simulink model "pool_task"  (Simulink 3.00)
libraries: logiclib x14, mathlib x13, genlib x2, execlib x2, timelib x1

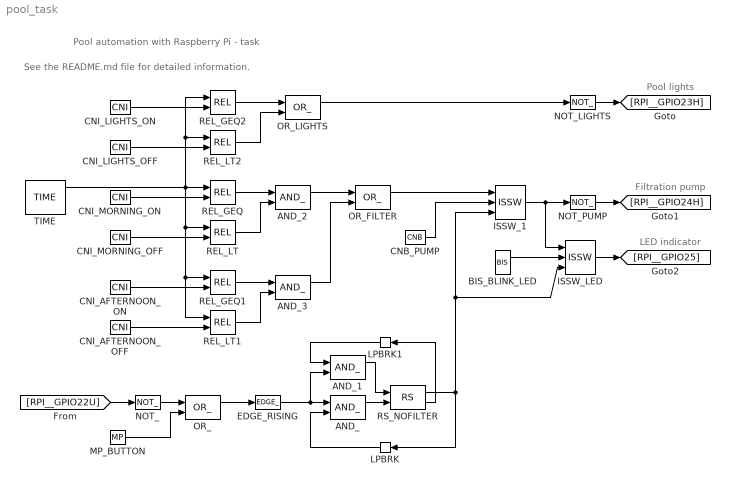
== system pool_task ==
  note: Pool lights
  note: Filtration pump
  note: LED indicator
  note: See the README.md file for detailed information.
  note: Pool automation with Raspberry Pi - task
  AND_{,1..3} (4 alike) : logiclib/AND_
  BIS_BLINK_LED : genlib/BIS  Y0=off  t1=0.1  t2=0.2  t3=0  t4=0  t5=0  t6=0  t7=2.0  t8=0  RPT=on  bEdit=off
  CNB_PUMP : mathlib/CNB  YCN=off
  CNI_AFTERNOON_OFF : mathlib/CNI  icn=14
  CNI_AFTERNOON_ON : mathlib/CNI  icn=13
  CNI_LIGHTS_OFF : mathlib/CNI  icn=1
  CNI_LIGHTS_ON : mathlib/CNI  icn=21
  CNI_MORNING_OFF : mathlib/CNI  icn=4
  CNI_MORNING_ON : mathlib/CNI  icn=2
  EDGE_RISING : logiclib/EDGE_  iedge=1: Rising edge
  ISSW_1 : logiclib/ISSW
  ISSW_LED : logiclib/ISSW
  LPBRK : execlib/LPBRK  Orientation=left
  LPBRK1 : execlib/LPBRK  Orientation=left
  MP_BUTTON : genlib/MP  pwidth=1  BSTATE=off  RPTF=off
  NOT_ : logiclib/NOT_
  NOT_LIGHTS : logiclib/NOT_
  NOT_PUMP : logiclib/NOT_
  OR_ : logiclib/OR_
  OR_FILTER : logiclib/OR_
  OR_LIGHTS : logiclib/OR_
  REL_GEQ : mathlib/REL  irel=6: greater or equal (>=)
  REL_GEQ1 : mathlib/REL  irel=6: greater or equal (>=)
  REL_GEQ2 : mathlib/REL  irel=6: greater or equal (>=)
  REL_LT : mathlib/REL  irel=3: less than (<)
  REL_LT1 : mathlib/REL  irel=3: less than (<)
  REL_LT2 : mathlib/REL  irel=3: less than (<)
  RS_NOFILTER : logiclib/RS
  TIME : timelib/TIME  tz=1: Local time
  wires:
  AND_/1 -> RS_NOFILTER/2
  AND_1/1 -> RS_NOFILTER/1
  AND_2/1 -> OR_FILTER/1
  AND_3/1 -> OR_FILTER/2
  BIS_BLINK_LED/1 -> ISSW_LED/2
  CNB_PUMP/1 -> ISSW_1/2
  CNI_AFTERNOON_OFF/1 -> REL_LT1/2
  CNI_AFTERNOON_ON/1 -> REL_GEQ1/2
  CNI_LIGHTS_OFF/1 -> REL_LT2/2
  CNI_LIGHTS_ON/1 -> REL_GEQ2/2
  CNI_MORNING_OFF/1 -> REL_LT/2
  CNI_MORNING_ON/1 -> REL_GEQ/2
  EDGE_RISING/1 -> AND_/1, AND_1/2
  [RPI__GPIO22U] -> NOT_/1
  ISSW_1/1 -> ISSW_LED/1, NOT_PUMP/1
  ISSW_LED/1 -> [RPI__GPIO25]
  LPBRK/1 -> AND_/2
  LPBRK1/1 -> AND_1/1
  MP_BUTTON/1 -> OR_/2
  NOT_/1 -> OR_/1
  NOT_LIGHTS/1 -> [RPI__GPIO23H]
  NOT_PUMP/1 -> [RPI__GPIO24H]
  OR_/1 -> EDGE_RISING/1
  OR_FILTER/1 -> ISSW_1/1
  OR_LIGHTS/1 -> NOT_LIGHTS/1
  REL_GEQ/1 -> AND_2/1
  REL_GEQ1/1 -> AND_3/1
  REL_GEQ2/1 -> OR_LIGHTS/1
  REL_LT/1 -> AND_2/2
  REL_LT1/1 -> AND_3/2
  REL_LT2/1 -> OR_LIGHTS/2
  RS_NOFILTER/1 -> LPBRK/1, ISSW_1/3, ISSW_LED/3
  RS_NOFILTER/2 -> LPBRK1/1
  TIME/1 -> REL_GEQ/1, REL_LT/1, REL_GEQ1/1, REL_LT1/1, REL_GEQ2/1, REL_LT2/1
